simulink model "JetStar_MIL_Simulink"  (R2024b)
settings: Solver=ode4  StartTime=0.0  StopTime=5000  FixedStep=T_Step  RelTol=1e-3
undefined symbols (not defined in the file or in its folder): A_Full_Linear_Long, A_lat, alpha, alpha_calc_rad, alpha_rad, B_Full_Linear_Long, B_lat, beta, beta_rad, C_Full_Linear_Long, C_lat, D_Full_Linear_Long, D_lat, deg, delta_aileron_action_rad, delta_beta_rad, delta_elevator_action_rad, delta_p_radsec, delta_phi_rad, delta_psi_rad, delta_q_radsec, delta_r_radsec, delta_rudder_action_rad, delta_theta_rad, delta_thrust_action_lbs, delta_u, delta_v, delta_w, Earth, ft, g, gamma_calc_rad, H_calc_ft, H_ft, initial, Ixx, Iyy, Izz, m, Matrix_Controls, Matrix_States, p, p_radsec, phi, phi_rad, psi, psi_rad, q, q_radsec, r, r_radsec, rad, RefStates, s, theta, theta_rad, v, V_total, Vehicle, Vtot ... (+9)
libraries: aerolibconvert2 x53, simulink_extras x10, dspsrcs4 x2, aerolibasang x2, aerolibfltsims x2, SignalEditorBlockLib x1, shared6dof x1, dspsigops x1, aerolibtransform2 x1
settings Model: Creator=Abdallah Saleh  LastModifiedBy=mosta

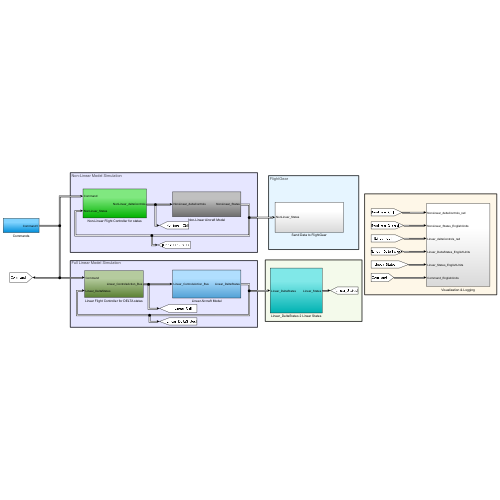
[thumbnail: Simulink's stored preview of the top-level diagram]
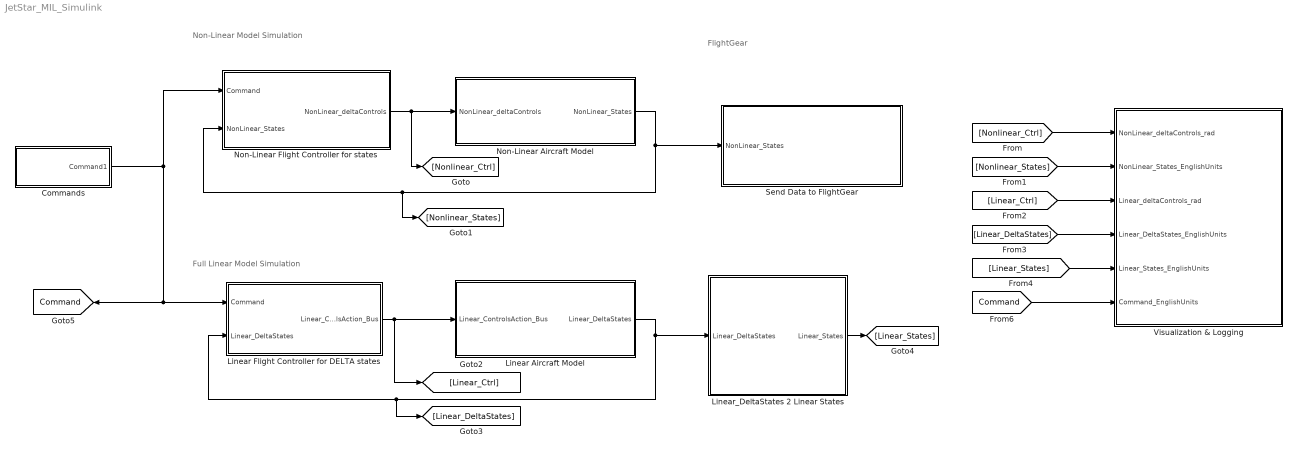
== system JetStar_MIL_Simulink ==
  note: FlightGear
  note: Non-Linear Model Simulation
  note: Full Linear Model Simulation
  Commands : Subsystem
  Linear Aircraft Model : Subsystem
  Linear Flight Controller for DELTA states : Subsystem
  Linear_DeltaStates 2 Linear States : Subsystem
  Non-Linear Aircraft Model : Subsystem
  Non-Linear Flight Controller for states : Subsystem
  Send Data to FlightGear : Subsystem
  Visualization & Logging : Subsystem
  tag scope: Command=global
  wires:
  Non-Linear Flight Controller for states/1(NonLinear_deltaControls) -> [Nonlinear_Ctrl], Non-Linear Aircraft Model/1(NonLinear_deltaControls)
  Non-Linear Aircraft Model/1(NonLinear_States) -> [Nonlinear_States], Non-Linear Flight Controller for states/2(NonLinear_States), Send Data to FlightGear/1(NonLinear_States)
  Linear Flight Controller for DELTA states/1(Linear_ControlsAction_Bus) -> [Linear_Ctrl], Linear Aircraft Model/1(Linear_ControlsAction_Bus)
  Linear Aircraft Model/1(Linear_DeltaStates) -> Linear Flight Controller for DELTA states/2(Linear_DeltaStates), [Linear_DeltaStates], Linear_DeltaStates 2 Linear States/1(Linear_DeltaStates)
  [Nonlinear_Ctrl] -> Visualization & Logging/1(NonLinear_deltaControls_rad)
  [Nonlinear_States] -> Visualization & Logging/2(NonLinear_States_EnglishUnits)
  [Linear_Ctrl] -> Visualization & Logging/3(Linear_deltaControls_rad)
  [Linear_DeltaStates] -> Visualization & Logging/4(Linear_DeltaStates_EnglishUnits)
  Linear_DeltaStates 2 Linear States/1(Linear_States) -> [Linear_States]
  [Linear_States] -> Visualization & Logging/5(Linear_States_EnglishUnits)
  [Command] -> Visualization & Logging/6(Command_EnglishUnits)
  Commands/1(Command1) -> Non-Linear Flight Controller for states/1(Command), Linear Flight Controller for DELTA states/1(Command), [Command]

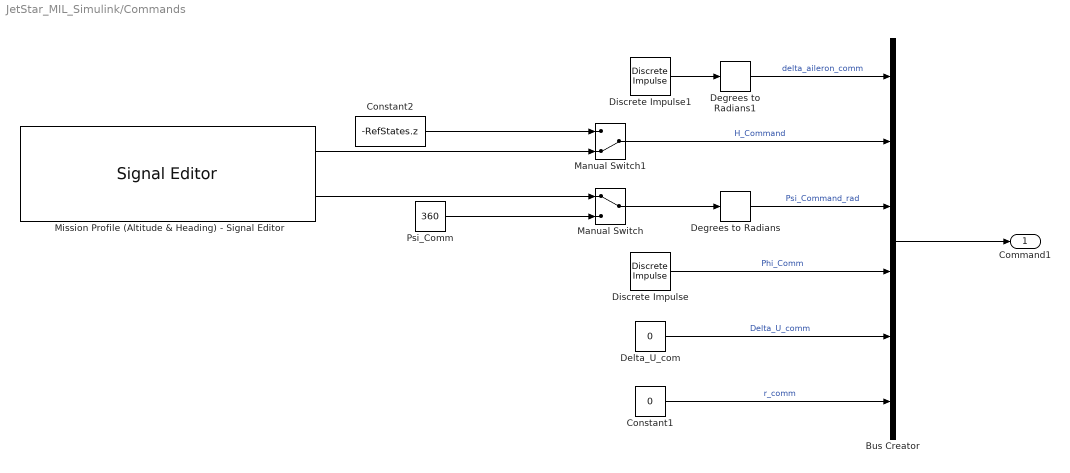
== system JetStar_MIL_Simulink/Commands ==
  Bus Creator : BusCreator  Inputs=6
  Constant1 : Constant  Value=0
  Constant2 : Constant  Value=-RefStates.z
  Degrees to Radians : simulink_extras/Transformations/Degrees to Radians
  Degrees to Radians1 : simulink_extras/Transformations/Degrees to Radians
  Delta_U_com : Constant  Value=0
  Discrete Impulse : dspsrcs4/Discrete  Impulse  Delay=2  SampleTime=15  FrameSample=1  OutputFrames=off  dataType=double  isSigned=on  wordLen=16  udDataType=sfix(16)  fracBitsMode=Best precision  numFracBits=15  OutDataTypeStr=double  LastOutDataTypeStr=double
  Discrete Impulse1 : dspsrcs4/Discrete  Impulse  Delay=1  SampleTime=3  FrameSample=1  OutputFrames=off  dataType=double  isSigned=on  wordLen=16  udDataType=sfix(16)  fracBitsMode=Best precision  numFracBits=15  OutDataTypeStr=double  LastOutDataTypeStr=double
  Manual Switch : ManualSwitch
  Manual Switch1 : ManualSwitch  CurrentSetting=0
  Mission Profile (Altitude & Heading) - Signal Editor : SignalEditorBlockLib/Signal Editor  FileName=Mission_Command.mat  ActiveScenario=Scenario  ActiveSignal=H_mission  IsBus=off  OutputBusObjectStr=Bus: BusObject  SampleTime=0  ZeroCross=off  OutputAfterFinalValue=Setting to zero  Unit=inherit  PreserveSignalName=on  ApplySigPropsToAllScenarios=off  ApplySigPropsToAllSignals=on
  Psi_Comm : Constant  Value=360
  Command1 : Outport
  wires:
  Constant1/1 -> Bus Creator/6  "r_comm"
  Manual Switch1/1 -> Bus Creator/2  "H_Command"
  Degrees to Radians/1 -> Bus Creator/3  "Psi_Command_rad"
  Delta_U_com/1 -> Bus Creator/5  "Delta_U_comm"
  Discrete Impulse/1 -> Bus Creator/4  "Phi_Comm"
  Psi_Comm/1 -> Manual Switch/2
  Manual Switch/1 -> Degrees to Radians/1
  Constant2/1 -> Manual Switch1/1
  Bus Creator/1 -> Command1/1
  Degrees to Radians1/1 -> Bus Creator/1  "delta_aileron_comm"
  Discrete Impulse1/1 -> Degrees to Radians1/1
  Mission Profile (Altitude & Heading) - Signal Editor/2 -> Manual Switch/1
  Mission Profile (Altitude & Heading) - Signal Editor/1 -> Manual Switch1/2

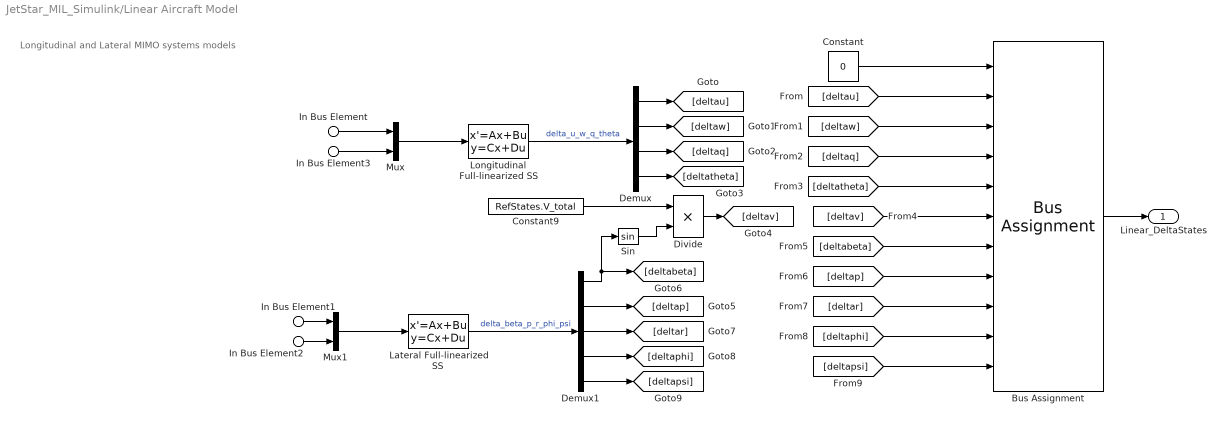
== system JetStar_MIL_Simulink/Linear Aircraft Model ==
  note: Longitudinal and Lateral MIMO systems models
  In Bus Element : Inport  PortName=Linear_ControlsAction_Bus  Element=delta_elevator_action_rad
  In Bus Element1 : Inport  PortName=Linear_ControlsAction_Bus  Element=delta_aileron_action_rad
  In Bus Element2 : Inport  PortName=Linear_ControlsAction_Bus  Element=delta_rudder_action_rad
  In Bus Element3 : Inport  PortName=Linear_ControlsAction_Bus  Element=delta_thrust_action_lbs
  Bus Assignment : BusAssignment  AssignedSignals=delta_u,delta_w,delta_q_radsec,delta_theta_rad,delta_v,delta_beta_rad,delta_p_radsec,delta_r_radsec,delta_phi_rad,delta_psi_rad
  Constant : Constant  Value=0  OutDataTypeStr=Bus: Linear_DeltaStates_Bus
  Constant9 : Constant  Value=RefStates.V_total
  Demux : Demux
  Demux1 : Demux  Outputs=5
  Divide : Product  Inputs=**
  Lateral Full-linearized SS : StateSpace  A=A_lat  B=B_lat  C=C_lat  D=D_lat  InitialCondition=0
  Longitudinal Full-linearized SS : StateSpace  A=A_Full_Linear_Long  B=B_Full_Linear_Long  C=C_Full_Linear_Long  D=D_Full_Linear_Long  InitialCondition=0
  Mux : Mux  Inputs=2
  Mux1 : Mux  Inputs=2
  Sin : Trigonometry
  Linear_DeltaStates : Outport  OutDataTypeStr=Bus: Linear_DeltaStates_Bus
  wires:
  In Bus Element/1 -> Mux/1
  Mux/1 -> Longitudinal Full-linearized SS/1
  In Bus Element3/1 -> Mux/2
  Longitudinal Full-linearized SS/1 -> Demux/1  "delta_u_w_q_theta"
  Mux1/1 -> Lateral Full-linearized SS/1
  Lateral Full-linearized SS/1 -> Demux1/1  "delta_beta_p_r_phi_psi"
  Demux1/1 -> [deltabeta], Sin/1
  In Bus Element2/1 -> Mux1/2
  In Bus Element1/1 -> Mux1/1
  Constant9/1 -> Divide/1
  Sin/1 -> Divide/2
  Constant/1 -> Bus Assignment/1
  Demux/1 -> [deltau]
  Demux/2 -> [deltaw]
  Demux/3 -> [deltaq]
  Demux/4 -> [deltatheta]
  Divide/1 -> [deltav]
  Demux1/2 -> [deltap]
  Demux1/3 -> [deltar]
  Demux1/4 -> [deltaphi]
  Demux1/5 -> [deltapsi]
  [deltau] -> Bus Assignment/2
  [deltaw] -> Bus Assignment/3
  [deltaq] -> Bus Assignment/4
  [deltatheta] -> Bus Assignment/5
  [deltav] -> Bus Assignment/6
  [deltabeta] -> Bus Assignment/7
  [deltap] -> Bus Assignment/8
  [deltar] -> Bus Assignment/9
  [deltaphi] -> Bus Assignment/10
  [deltapsi] -> Bus Assignment/11
  Bus Assignment/1 -> Linear_DeltaStates/1

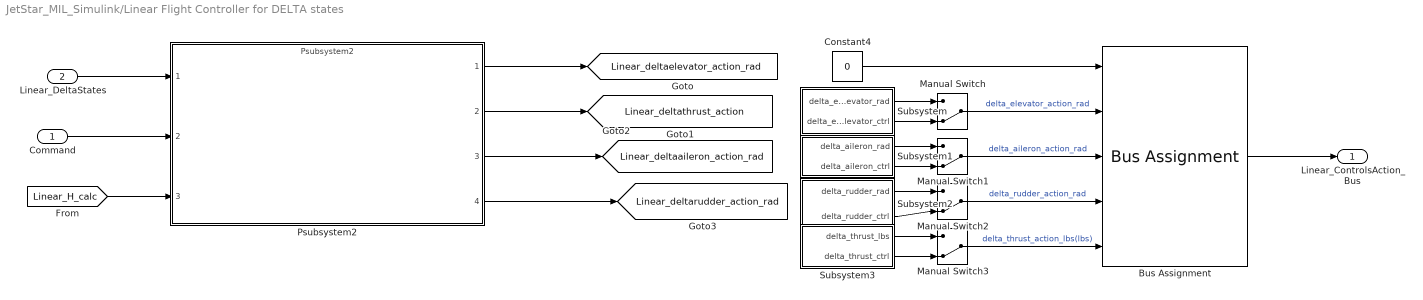
== system JetStar_MIL_Simulink/Linear Flight Controller for DELTA states ==
  Command : Inport
  Linear_DeltaStates : Inport  Port=2
  Bus Assignment : BusAssignment  AssignedSignals=delta_elevator_action_rad,delta_aileron_action_rad,delta_rudder_action_rad,delta_thrust_action_lbs
  Constant4 : Constant  Value=0  OutDataTypeStr=Bus: Linear_ControlsAction_Bus
  Manual Switch{,1..3} (4 alike) : ManualSwitch  CurrentSetting=0
  Psubsystem2 : ModelReference  ModelNameDialog=Psubsystem2  ModelReferenceVersion=1.395  CopyOfModelProtected=on
  Subsystem : Subsystem
  Subsystem1 : Subsystem
  Subsystem2 : Subsystem
  Subsystem3 : Subsystem
  Linear_ControlsAction_Bus : Outport  OutDataTypeStr=Bus: Linear_ControlsAction_Bus
  tag scope: Linear_deltaaileron_action_rad=global, Linear_deltaelevator_action_rad=global, Linear_deltarudder_action_rad=global, Linear_deltathrust_action=global
  wires:
  Constant4/1 -> Bus Assignment/1
  Manual Switch/1 -> Bus Assignment/2  "delta_elevator_action_rad"
  Manual Switch1/1 -> Bus Assignment/3  "delta_aileron_action_rad"
  Manual Switch2/1 -> Bus Assignment/4  "delta_rudder_action_rad"
  Manual Switch3/1 -> Bus Assignment/5  "delta_thrust_action_lbs(lbs)"
  Bus Assignment/1 -> Linear_ControlsAction_Bus/1
  Subsystem/1(delta_elevator_rad) -> Manual Switch/1
  Subsystem/2(delta_elevator_ctrl) -> Manual Switch/2
  Subsystem1/1(delta_aileron_rad) -> Manual Switch1/1
  Subsystem1/2(delta_aileron_ctrl) -> Manual Switch1/2
  Subsystem2/1(delta_rudder_rad) -> Manual Switch2/1
  Subsystem2/2(delta_rudder_ctrl) -> Manual Switch2/2
  Subsystem3/1(delta_thrust_lbs) -> Manual Switch3/1
  Subsystem3/2(delta_thrust_ctrl) -> Manual Switch3/2
  Linear_DeltaStates/1 -> Psubsystem2/1
  [Linear_H_calc] -> Psubsystem2/3
  Command/1 -> Psubsystem2/2
  Psubsystem2/1 -> [Linear_deltaelevator_action_rad]
  Psubsystem2/2 -> [Linear_deltathrust_action]
  Psubsystem2/3 -> [Linear_deltaaileron_action_rad]
  Psubsystem2/4 -> [Linear_deltarudder_action_rad]

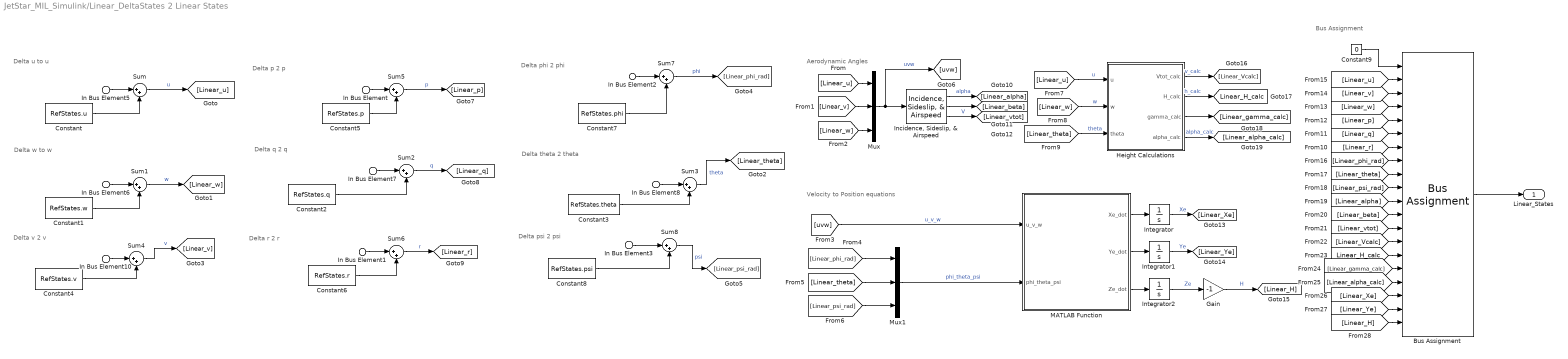
== system JetStar_MIL_Simulink/Linear_DeltaStates 2 Linear States ==
  note: Bus Assignment
  note: Velocity to Position equations
  note: Aerodynamic Angles
  note: Delta psi 2 psi
  note: Delta phi 2 phi
  note: Delta r 2 r
  note: Delta p 2 p
  note: Delta v 2 v
  note: Delta theta 2 theta
  note: Delta q 2 q
  note: Delta w to w
  note: Delta u to u
  In Bus Element : Inport  PortName=Linear_DeltaStates  Element=delta_p_radsec
  In Bus Element1 : Inport  PortName=Linear_DeltaStates  Element=delta_r_radsec
  In Bus Element2 : Inport  PortName=Linear_DeltaStates  Element=delta_phi_rad
  In Bus Element3 : Inport  PortName=Linear_DeltaStates  Element=delta_psi_rad
  In Bus Element5 : Inport  PortName=Linear_DeltaStates  Element=delta_u
  In Bus Element6 : Inport  PortName=Linear_DeltaStates  Element=delta_w
  In Bus Element7 : Inport  PortName=Linear_DeltaStates  Element=delta_q_radsec
  In Bus Element8 : Inport  PortName=Linear_DeltaStates  Element=delta_theta_rad
  In Bus Element10 : Inport  PortName=Linear_DeltaStates  Element=delta_v
  Bus Assignment : BusAssignment  AssignedSignals=u,v,w,p_radsec,q_radsec,r_radsec,phi_rad,theta_rad,psi_rad,alpha_rad,beta_rad,Vtot,Vtot_calc,H_calc_ft,gamma_calc_rad,alpha_calc_rad,Xe_ft,Ye_ft,H_ft
  Constant : Constant  Value=RefStates.u
  Constant1 : Constant  Value=RefStates.w
  Constant2 : Constant  Value=RefStates.q
  Constant3 : Constant  Value=RefStates.theta
  Constant4 : Constant  Value=RefStates.v
  Constant5 : Constant  Value=RefStates.p
  Constant6 : Constant  Value=RefStates.r
  Constant7 : Constant  Value=RefStates.phi
  Constant8 : Constant  Value=RefStates.psi
  Constant9 : Constant  Value=0  OutDataTypeStr=Bus: Linear_States_Bus
  Gain : Gain  Gain=-1
  Height Calculations : Subsystem
  "Incidence, Sideslip, & Airspeed" : aerolibasang/Incidence, Sideslip, & Airspeed
  Integrator : Integrator
  Integrator1 : Integrator
  Integrator2 : Integrator
  MATLAB Function : MATLAB Function  TreatAsAtomicUnit=on
  Mux : Mux  Inputs=3
  Mux1 : Mux  Inputs=3
  Sum{,1..8} (9 alike) : Sum  Inputs=|++
  Linear_States : Outport  OutDataTypeStr=Bus: Linear_States_Bus
  tag scope: Linear_H_calc=global
  wires:
  In Bus Element5/1 -> Sum/1
  Constant/1 -> Sum/2
  Sum/1 -> [Linear_u]  "u"
  In Bus Element6/1 -> Sum1/1
  Constant1/1 -> Sum1/2
  Sum1/1 -> [Linear_w]  "w"
  In Bus Element7/1 -> Sum2/1
  Constant2/1 -> Sum2/2
  Sum2/1 -> [Linear_q]  "q"
  In Bus Element8/1 -> Sum3/1
  Constant3/1 -> Sum3/2
  Sum3/1 -> [Linear_theta]  "theta"
  Constant4/1 -> Sum4/2
  Sum4/1 -> [Linear_v]  "v"
  In Bus Element/1 -> Sum5/1
  Constant5/1 -> Sum5/2
  Sum5/1 -> [Linear_p]  "p"
  In Bus Element1/1 -> Sum6/1
  Sum6/1 -> [Linear_r]  "r"
  Constant6/1 -> Sum6/2
  In Bus Element2/1 -> Sum7/1
  Constant7/1 -> Sum7/2
  Sum7/1 -> [Linear_phi_rad]  "phi"
  In Bus Element3/1 -> Sum8/1
  Constant8/1 -> Sum8/2
  Sum8/1 -> [Linear_psi_rad]  "psi"
  Mux/1 -> [uvw], "Incidence, Sideslip, & Airspeed"/1  "uvw"
  [Linear_u] -> Mux/1
  [Linear_v] -> Mux/2
  [Linear_w] -> Mux/3
  [Linear_phi_rad] -> Mux1/1
  [Linear_theta] -> Mux1/2
  [Linear_psi_rad] -> Mux1/3
  Mux1/1 -> MATLAB Function/2(phi_theta_psi)  "phi_theta_psi"
  In Bus Element10/1 -> Sum4/1
  [uvw] -> MATLAB Function/1(u_v_w)  "u_v_w"
  MATLAB Function/1(Xe_dot) -> Integrator/1
  MATLAB Function/2(Ye_dot) -> Integrator1/1
  MATLAB Function/3(Ze_dot) -> Integrator2/1
  Integrator2/1 -> Gain/1  "Ze"
  Gain/1 -> [Linear_H]  "H"
  [Linear_u] -> Height Calculations/1(u)  "u"
  [Linear_w] -> Height Calculations/2(w)  "w"
  [Linear_theta] -> Height Calculations/3(theta)  "theta"
  Height Calculations/1(Vtot_calc) -> [Linear_Vcalc]  "v_calc"
  Height Calculations/2(H_calc) -> [Linear_H_calc]  "h_calc"
  Height Calculations/3(gamma_calc) -> [Linear_gamma_calc]
  "Incidence, Sideslip, & Airspeed"/1 -> [Linear_alpha]  "alpha"
  "Incidence, Sideslip, & Airspeed"/2 -> [Linear_beta]
  "Incidence, Sideslip, & Airspeed"/3 -> [Linear_vtot]  "V"
  Integrator/1 -> [Linear_Xe]  "Xe"
  Integrator1/1 -> [Linear_Ye]  "Ye"
  Height Calculations/4(alpha_calc) -> [Linear_alpha_calc]  "alpha_calc"
  [Linear_u] -> Bus Assignment/2
  [Linear_v] -> Bus Assignment/3
  [Linear_w] -> Bus Assignment/4
  [Linear_p] -> Bus Assignment/5
  [Linear_q] -> Bus Assignment/6
  [Linear_r] -> Bus Assignment/7
  [Linear_phi_rad] -> Bus Assignment/8
  [Linear_theta] -> Bus Assignment/9
  [Linear_psi_rad] -> Bus Assignment/10
  [Linear_alpha] -> Bus Assignment/11
  [Linear_beta] -> Bus Assignment/12
  [Linear_vtot] -> Bus Assignment/13
  [Linear_Vcalc] -> Bus Assignment/14
  [Linear_H_calc] -> Bus Assignment/15
  [Linear_Xe] -> Bus Assignment/18
  [Linear_Ye] -> Bus Assignment/19
  [Linear_H] -> Bus Assignment/20
  [Linear_gamma_calc] -> Bus Assignment/16
  [Linear_alpha_calc] -> Bus Assignment/17
  Constant9/1 -> Bus Assignment/1
  Bus Assignment/1 -> Linear_States/1

== system JetStar_MIL_Simulink/Non-Linear Aircraft Model ==
  NonLinear_deltaControls : Inport  OutDataTypeStr=Bus: Nonlinear_ControlsAction_Bus
  Airframe_Model : Subsystem
  Delay1 : Delay  DelayLength=1  InitialCondition=RefStates
  Euler_6DOF : Subsystem
  NonLinear_States : Outport  OutDataTypeStr=Bus: Nonlinear_States_Bus
  wires:
  NonLinear_deltaControls/1 -> Airframe_Model/2(NonLinear_deltaControls)
  Delay1/1 -> Airframe_Model/1(StatesBus)
  Airframe_Model/1(Forces) -> Euler_6DOF/1(Forces)
  Airframe_Model/2(Moments) -> Euler_6DOF/2(Moments)
  Euler_6DOF/1(States) -> Delay1/1, NonLinear_States/1

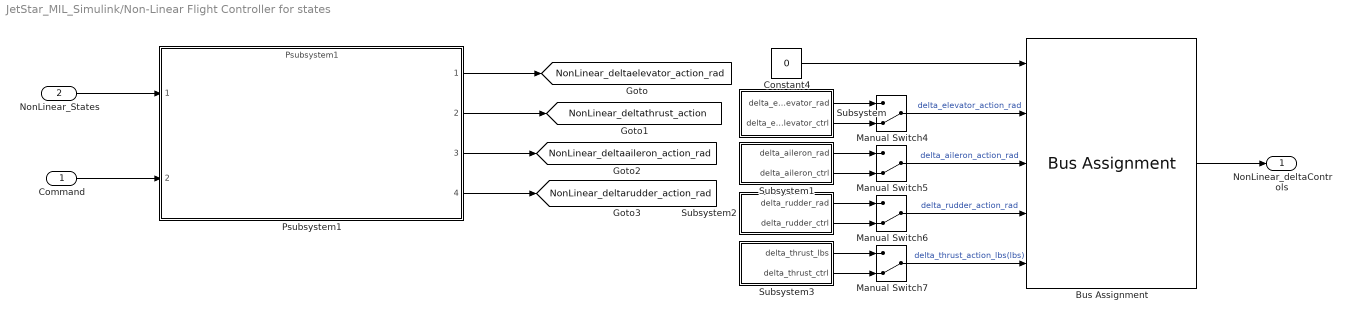
== system JetStar_MIL_Simulink/Non-Linear Flight Controller for states ==
  Command : Inport
  NonLinear_States : Inport  Port=2
  Bus Assignment : BusAssignment  AssignedSignals=delta_elevator_action_rad,delta_aileron_action_rad,delta_rudder_action_rad,delta_thrust_action_lbs
  Constant4 : Constant  Value=0  OutDataTypeStr=Bus: Nonlinear_ControlsAction_Bus
  Manual Switch{4..7} (4 alike) : ManualSwitch  CurrentSetting=0
  Psubsystem1 : ModelReference  ModelNameDialog=Psubsystem1  ModelReferenceVersion=1.395  CopyOfModelProtected=on
  Subsystem : Subsystem
  Subsystem1 : Subsystem
  Subsystem2 : Subsystem
  Subsystem3 : Subsystem
  NonLinear_deltaControls : Outport  OutDataTypeStr=Bus: Nonlinear_ControlsAction_Bus
  tag scope: NonLinear_deltaaileron_action_rad=global, NonLinear_deltaelevator_action_rad=global, NonLinear_deltarudder_action_rad=global, NonLinear_deltathrust_action=global
  wires:
  Constant4/1 -> Bus Assignment/1
  Bus Assignment/1 -> NonLinear_deltaControls/1
  Subsystem2/1(delta_rudder_rad) -> Manual Switch6/1
  Subsystem2/2(delta_rudder_ctrl) -> Manual Switch6/2
  Subsystem3/1(delta_thrust_lbs) -> Manual Switch7/1
  Subsystem3/2(delta_thrust_ctrl) -> Manual Switch7/2
  Subsystem/2(delta_elevator_ctrl) -> Manual Switch4/2
  Subsystem/1(delta_elevator_rad) -> Manual Switch4/1
  Subsystem1/2(delta_aileron_ctrl) -> Manual Switch5/2
  Manual Switch6/1 -> Bus Assignment/4  "delta_rudder_action_rad"
  Manual Switch5/1 -> Bus Assignment/3  "delta_aileron_action_rad"
  Manual Switch7/1 -> Bus Assignment/5  "delta_thrust_action_lbs(lbs)"
  Manual Switch4/1 -> Bus Assignment/2  "delta_elevator_action_rad"
  Subsystem1/1(delta_aileron_rad) -> Manual Switch5/1
  NonLinear_States/1 -> Psubsystem1/1
  Command/1 -> Psubsystem1/2
  Psubsystem1/1 -> [NonLinear_deltaelevator_action_rad]
  Psubsystem1/2 -> [NonLinear_deltathrust_action]
  Psubsystem1/3 -> [NonLinear_deltaaileron_action_rad]
  Psubsystem1/4 -> [NonLinear_deltarudder_action_rad]

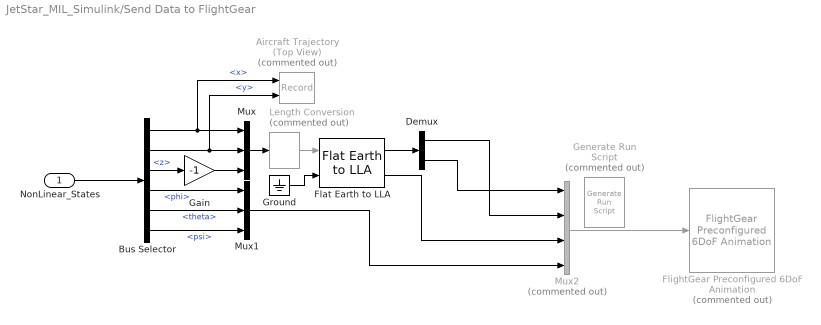
== system JetStar_MIL_Simulink/Send Data to FlightGear ==
  NonLinear_States : Inport  OutDataTypeStr=Bus: Nonlinear_States_Bus
  Aircraft Trajectory (Top View) : Record  Commented=on  FileSettingsInternal="{\"entries\":[{\"content\":{\"excelSettings\":{\"content\":{},\"type\":\"Streamout.ExcelSettings\"}},\"type\":\"Streamout.FileSettingStorage\",\"uuid\":\"\"}],\"packageUris\":[\"http:\\/\\/schema.mathworks.com\\/mf0\\/streamout_blocks\\/R2020a\"],\"version\":\"1.0\"}"  Layout=[1 1]  SignalsInternal="{\"entries\":[{\"content\":{},\"type\":\"RecordBlkView.InputSignals\",\"uuid\":\"\"}],\"packageUris\":[\"http:\\/\\/schema.mathworks.com\\/mf0\\/streamout_blocks\\/R2020a\"],\"version\":\"1.0\"}"  VisualizationBindings="{\"xyplotplugin\":{\"info\":[{\"series\":[],\"subplotID\":1}]}}"  CompatibilityTag=XY
  Bus Selector : BusSelector  OutputSignals=x,y,z,phi,theta,psi
  Demux : Demux  Outputs=2
  Flat Earth to LLA : aerolibtransform2/Flat Earth to LLA  units=Metric (MKS)  ptype=Earth (WGS84)  F=1/298.257223563  R=6378137  refPosPort=off  LL0=[0 10]  psi=0
  FlightGear Preconfigured 6DoF Animation : aerolibfltsims/FlightGear Preconfigured 6DoF Animation  Commented=on  xFlightGearVersion=v2019.1  DestinationIpAddress=127.0.0.1  DestinationPort=5502  SampleTime=-1  packetVersion=24
  Gain : Gain  Gain=-1
  Generate Run Script : aerolibfltsims/Generate Run Script  Commented=on  Architecture=Win64  dataFlow=Send  GeometryModelName=HL20  AirportId=KSFO  RunwayId=10L  InitialAltitude=0  InitialHeading=0  OffsetDistance=0  OffsetAzimuth=0  InstallScenery=off  DisableShaders=on  OriginAddress=127.0.0.1  DestinationPort=5502  OriginPort=5505  LocalAddress=127.0.0.1  OutputFileName=runfg.bat  FlightGearBaseDirectory=C:\Program Files\FlightGear 2024.1
  Ground : Ground
  Length Conversion : aerolibconvert2/Length Conversion  Commented=on  IU=ft  OU=m
  Mux : Mux  Inputs=3
  Mux1 : Mux  Inputs=3
  Mux2 : Mux  Commented=on
  wires:
  NonLinear_States/1 -> Bus Selector/1
  Bus Selector/1 -> Mux/1, Aircraft Trajectory (Top View)/1  "<x>"
  Bus Selector/2 -> Mux/2, Aircraft Trajectory (Top View)/2  "<y>"
  Bus Selector/3 -> Gain/1  "<z>"
  Bus Selector/4 -> Mux1/1  "<phi>"
  Bus Selector/5 -> Mux1/2  "<theta>"
  Bus Selector/6 -> Mux1/3  "<psi>"
  Mux/1 -> Length Conversion/1
  Ground/1 -> Flat Earth to LLA/2
  Mux2/1 -> FlightGear Preconfigured 6DoF Animation/1
  Flat Earth to LLA/1 -> Demux/1
  Demux/1 -> Mux2/2
  Demux/2 -> Mux2/1
  Mux1/1 -> Mux2/4
  Flat Earth to LLA/2 -> Mux2/3
  Length Conversion/1 -> Flat Earth to LLA/1
  Gain/1 -> Mux/3

== system JetStar_MIL_Simulink/Visualization & Logging ==
  NonLinear_deltaControls_rad : Inport
  NonLinear_States_EnglishUnits : Inport  Port=2
  Linear_deltaControls_rad : Inport  Port=3
  Linear_DeltaStates_EnglishUnits : Inport  Port=4
  Linear_States_EnglishUnits : Inport  Port=5
  Command_EnglishUnits : Inport  Port=6
  Units conversion & Data logging : Subsystem
  Units conversion & Data logging1 : Subsystem
  Units conversion & Data logging2 : Subsystem
  Units conversion & Data logging3 : Subsystem
  Units conversion & Data logging4 : Subsystem
  Units conversion & Data logging5 : Subsystem
  wires:
  NonLinear_States_EnglishUnits/1 -> Units conversion & Data logging1/1(NonLinear_States_EnglishUnits)  "NonLinear_States_EnglishUnits"
  Linear_deltaControls_rad/1 -> Units conversion & Data logging2/1(Linear_deltaControls_rad)  "Linear_deltaControls_rad"
  Linear_DeltaStates_EnglishUnits/1 -> Units conversion & Data logging3/1(Linear_DeltaStates_EnglishUnits)  "Linear_DeltaStates_EnglishUnits"
  Linear_States_EnglishUnits/1 -> Units conversion & Data logging4/1(Linear_States_EnglishUnits)  "Linear_States_EnglishUnits"
  NonLinear_deltaControls_rad/1 -> Units conversion & Data logging/1(NonLinear_deltaControls_rad)  "NonLinear_deltaControls_rad"
  Command_EnglishUnits/1 -> Units conversion & Data logging5/1(Command_EnglishUnits)  "Command_EnglishUnits"

== system JetStar_MIL_Simulink/Linear Flight Controller for DELTA states/Subsystem ==
  Constant : Constant  Value=0
  Degrees to Radians : simulink_extras/Transformations/Degrees to Radians
  delta_elevator_rad : Outport
  delta_elevator_ctrl : Outport  Port=2
  wires:
  [Linear_deltaelevator_action_rad] -> delta_elevator_ctrl/1  "delta_elevator_ctrl"
  Constant/1 -> Degrees to Radians/1
  Degrees to Radians/1 -> delta_elevator_rad/1  "delta_elevator_rad"

== system JetStar_MIL_Simulink/Linear Flight Controller for DELTA states/Subsystem1 ==
  Constant1 : Constant  Value=0
  Degrees to Radians1 : simulink_extras/Transformations/Degrees to Radians
  delta_aileron_rad : Outport
  delta_aileron_ctrl : Outport  Port=2
  wires:
  Constant1/1 -> Degrees to Radians1/1
  [Linear_deltaaileron_action_rad] -> delta_aileron_ctrl/1  "delta_aileron_ctrl"
  Degrees to Radians1/1 -> delta_aileron_rad/1  "delta_aileron_rad"

== system JetStar_MIL_Simulink/Linear Flight Controller for DELTA states/Subsystem2 ==
  Constant2 : Constant  Value=0
  Degrees to Radians2 : simulink_extras/Transformations/Degrees to Radians
  delta_rudder_rad : Outport
  delta_rudder_ctrl : Outport  Port=2
  wires:
  Constant2/1 -> Degrees to Radians2/1
  [Linear_deltarudder_action_rad] -> delta_rudder_ctrl/1  "delta_rudder_ctrl"
  Degrees to Radians2/1 -> delta_rudder_rad/1  "delta_rudder_rad"

== system JetStar_MIL_Simulink/Linear Flight Controller for DELTA states/Subsystem3 ==
  Constant3 : Constant  Value=0
  delta_thrust_lbs : Outport
  delta_thrust_ctrl : Outport  Port=2
  wires:
  [Linear_deltathrust_action] -> delta_thrust_ctrl/1  "delta_thrust_ctrl"
  Constant3/1 -> delta_thrust_lbs/1  "delta_thrust_lbs"

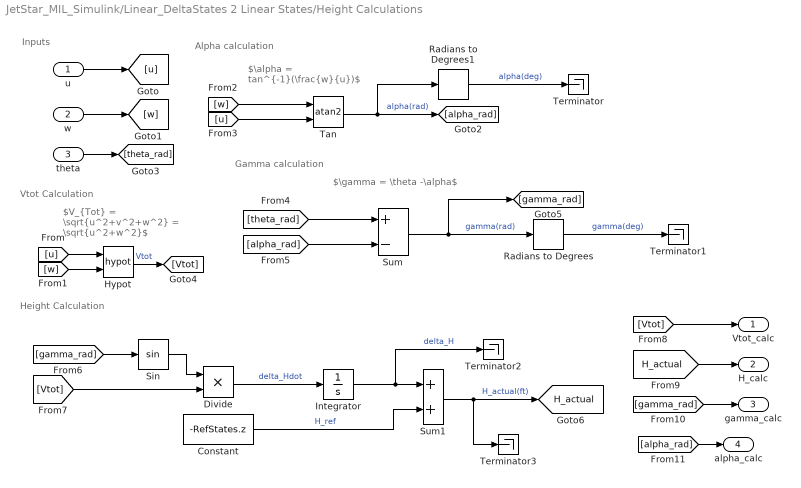
== system JetStar_MIL_Simulink/Linear_DeltaStates 2 Linear States/Height Calculations ==
  note: Gamma calculation
  note: $\alpha = tan^{-1}(\frac{w}{u})$
  note: Alpha calculation
  note: Inputs
  note: Height Calculation
  note: $V_{Tot} = \sqrt{u^2+v^2+w^2} = \sqrt{u^2+w^2}$
  note: $\gamma = \theta -\alpha$
  note: Vtot Calculation
  u : Inport
  w : Inport  Port=2
  theta : Inport  Port=3
  Constant : Constant  Value=-RefStates.z
  Divide : Product  Inputs=**
  Hypot : Math  Operator=hypot
  Integrator : Integrator
  Radians to Degrees : simulink_extras/Transformations/Radians to Degrees
  Radians to Degrees1 : simulink_extras/Transformations/Radians to Degrees
  Sin : Trigonometry
  Sum : Sum  Inputs=+-
  Sum1 : Sum
  Tan : Trigonometry  Operator=atan2
  Terminator{,1..3} (4 alike) : Terminator
  Vtot_calc : Outport
  H_calc : Outport  Port=2
  gamma_calc : Outport  Port=3
  alpha_calc : Outport  Port=4
  tag scope: H_actual=global
  wires:
  Sum/1 -> [gamma_rad], Radians to Degrees/1  "gamma(rad)"
  Sum1/1 -> Terminator3/1, [H_actual]  "H_actual(ft)"
  Hypot/1 -> [Vtot]  "Vtot"
  [theta_rad] -> Sum/1
  [u] -> Tan/2
  Constant/1 -> Sum1/2  "H_ref"
  Divide/1 -> Integrator/1  "delta_Hdot"
  [u] -> Hypot/1
  theta/1 -> [theta_rad]
  [Vtot] -> Divide/2
  Tan/1 -> Radians to Degrees1/1, [alpha_rad]  "alpha(rad)"
  [gamma_rad] -> Sin/1
  Radians to Degrees/1 -> Terminator1/1  "gamma(deg)"
  Integrator/1 -> Terminator2/1, Sum1/1  "delta_H"
  Sin/1 -> Divide/1
  [w] -> Tan/1
  [alpha_rad] -> Sum/2
  [w] -> Hypot/2
  u/1 -> [u]
  w/1 -> [w]
  Radians to Degrees1/1 -> Terminator/1  "alpha(deg)"
  [Vtot] -> Vtot_calc/1
  [H_actual] -> H_calc/1
  [gamma_rad] -> gamma_calc/1
  [alpha_rad] -> alpha_calc/1

== system JetStar_MIL_Simulink/Non-Linear Aircraft Model/Airframe_Model ==
  StatesBus : Inport
  NonLinear_deltaControls : Inport  Port=2
  Deltas Forces and Moments : Subsystem
  "Intertias gain " : Gain  Gain=[Ixx;Iyy;Izz]
  "Mass gain " : Gain  Gain=Vehicle.Airframe.mass
  ReferenceForces : Constant  Value=initial.forces  VectorParams1D=off
  ReferenceMoments : Constant  Value=initial.moments
  Sum : Sum  Inputs=|++
  "Sum " : Sum
  Forces : Outport
  Moments : Outport  Port=2
  wires:
  ReferenceMoments/1 -> Sum/2
  Deltas Forces and Moments/2(DeltaMoments) -> "Intertias gain "/1
  Deltas Forces and Moments/1(DeltaForces) -> "Mass gain "/1
  StatesBus/1 -> Deltas Forces and Moments/1(StatesBus)
  Sum/1 -> Moments/1
  ReferenceForces/1 -> "Sum "/1
  "Intertias gain "/1 -> Sum/1
  "Mass gain "/1 -> "Sum "/2
  NonLinear_deltaControls/1 -> Deltas Forces and Moments/2(NonLinear_deltaControls)
  "Sum "/1 -> Forces/1

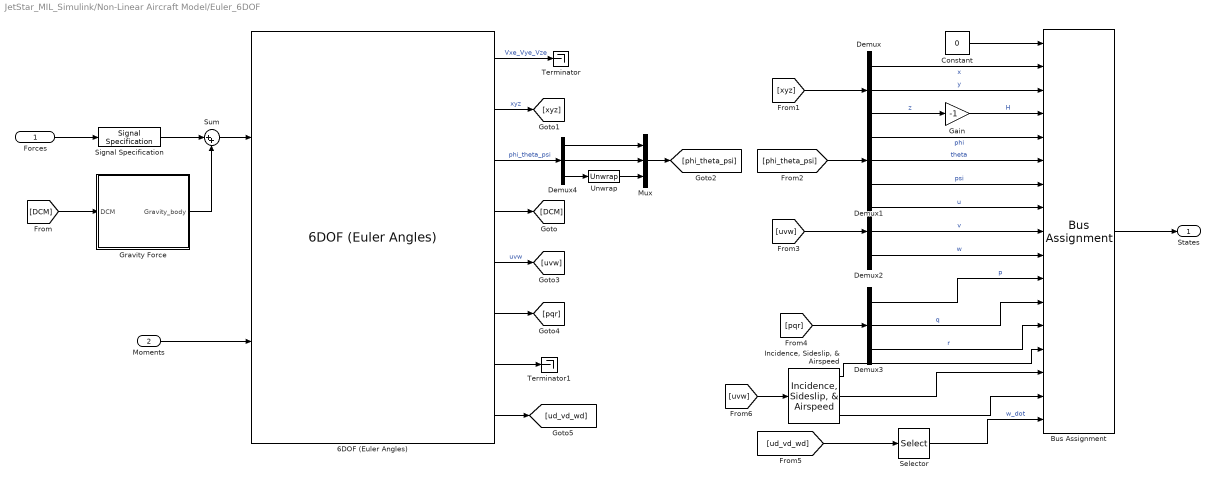
== system JetStar_MIL_Simulink/Non-Linear Aircraft Model/Euler_6DOF ==
  Forces : Inport
  Moments : Inport  Port=2
  6DOF (Euler Angles) : shared6dof/6DOF (Euler Angles)  units=English (Velocity in ft/s)  mtype=Fixed  rep=Euler Angles  xme_0=initial.position  Vm_0=initial.Vbody  eul_0=initial.Euler_Angles  pm_0=initial.AngRates  mass_0=Vehicle.Airframe.mass  mass_e=0.5  mass_f=2.0  inertia=Vehicle.Airframe.inertias  inertia_e=eye(3)  inertia_f=2*eye(3)  k_quat=1.0  vre_flag=on  abi_flag=off  aMode=0  xme_statename=''  Vm_statename=''  eul_statename=''  quat_statename=''  pm_statename=''  mass_statename=''
  Bus Assignment : BusAssignment  AssignedSignals=x,y,z,phi,theta,psi,u,v,w,p,q,r,alpha,beta,V_total,w_dot
  Constant : Constant  Value=0  OutDataTypeStr=Bus: Nonlinear_States_Bus
  Demux{,1..4} (5 alike) : Demux  Outputs=3
  Gain : Gain  Gain=-1
  Gravity Force : Subsystem
  "Incidence, Sideslip, & Airspeed" : aerolibasang/Incidence, Sideslip, & Airspeed
  Mux : Mux  Inputs=3
  Selector : Selector  InputPortWidth=3  IndexOptions=Index vector (dialog)  Indices=[3]  OutputSizes=1
  Signal Specification : SignalSpecification  Dimensions=[3 1]
  Sum : Sum  Inputs=|++
  Terminator : Terminator
  Terminator1 : Terminator
  Unwrap : dspsigops/Unwrap  tol=pi  InputProcessing=Columns as channels (frame based)  running=off
  States : Outport  OutDataTypeStr=Bus: Nonlinear_States_Bus
  wires:
  6DOF (Euler Angles)/8 -> [ud_vd_wd]
  6DOF (Euler Angles)/4 -> [DCM]
  Constant/1 -> Bus Assignment/1
  Moments/1 -> 6DOF (Euler Angles)/2
  Bus Assignment/1 -> States/1
  6DOF (Euler Angles)/1 -> Terminator/1  "Vxe_Vye_Vze"
  6DOF (Euler Angles)/2 -> [xyz]  "xyz"
  [xyz] -> Demux/1
  Demux/1 -> Bus Assignment/2  "x"
  Demux/2 -> Bus Assignment/3  "y"
  Demux/3 -> Gain/1  "z"
  [phi_theta_psi] -> Demux1/1
  Demux1/1 -> Bus Assignment/5  "phi"
  Demux1/2 -> Bus Assignment/6  "theta"
  Demux1/3 -> Bus Assignment/7  "psi"
  Demux2/1 -> Bus Assignment/8  "u"
  Demux2/2 -> Bus Assignment/9  "v"
  6DOF (Euler Angles)/5 -> [uvw]  "uvw"
  [uvw] -> Demux2/1
  6DOF (Euler Angles)/6 -> [pqr]
  [pqr] -> Demux3/1
  6DOF (Euler Angles)/7 -> Terminator1/1
  [uvw] -> "Incidence, Sideslip, & Airspeed"/1
  [ud_vd_wd] -> Selector/1
  [DCM] -> Gravity Force/1(DCM)
  Sum/1 -> 6DOF (Euler Angles)/1
  Forces/1 -> Signal Specification/1
  Gravity Force/1(Gravity_body) -> Sum/2
  Signal Specification/1 -> Sum/1
  Demux2/3 -> Bus Assignment/10  "w"
  Demux3/1 -> Bus Assignment/11  "p"
  Demux3/2 -> Bus Assignment/12  "q"
  Demux3/3 -> Bus Assignment/13  "r"
  "Incidence, Sideslip, & Airspeed"/1 -> Bus Assignment/14
  "Incidence, Sideslip, & Airspeed"/2 -> Bus Assignment/15
  "Incidence, Sideslip, & Airspeed"/3 -> Bus Assignment/16
  Selector/1 -> Bus Assignment/17  "w_dot"
  Gain/1 -> Bus Assignment/4  "H"
  6DOF (Euler Angles)/3 -> Demux4/1  "phi_theta_psi"
  Demux4/3 -> Unwrap/1
  Demux4/1 -> Mux/1
  Demux4/2 -> Mux/2
  Unwrap/1 -> Mux/3
  Mux/1 -> [phi_theta_psi]

== system JetStar_MIL_Simulink/Non-Linear Flight Controller for states/Subsystem ==
  Constant : Constant  Value=0
  Degrees to Radians : simulink_extras/Transformations/Degrees to Radians
  delta_elevator_rad : Outport
  delta_elevator_ctrl : Outport  Port=2
  wires:
  [NonLinear_deltaelevator_action_rad] -> delta_elevator_ctrl/1  "delta_elevator_ctrl"
  Constant/1 -> Degrees to Radians/1
  Degrees to Radians/1 -> delta_elevator_rad/1  "delta_elevator_rad"

== system JetStar_MIL_Simulink/Non-Linear Flight Controller for states/Subsystem1 ==
  Constant1 : Constant  Value=0
  Degrees to Radians1 : simulink_extras/Transformations/Degrees to Radians
  delta_aileron_rad : Outport
  delta_aileron_ctrl : Outport  Port=2
  wires:
  Constant1/1 -> Degrees to Radians1/1
  [NonLinear_deltaaileron_action_rad] -> delta_aileron_ctrl/1  "delta_aileron_ctrl"
  Degrees to Radians1/1 -> delta_aileron_rad/1  "delta_aileron_rad"

== system JetStar_MIL_Simulink/Non-Linear Flight Controller for states/Subsystem2 ==
  Constant2 : Constant  Value=0
  Degrees to Radians2 : simulink_extras/Transformations/Degrees to Radians
  delta_rudder_rad : Outport
  delta_rudder_ctrl : Outport  Port=2
  wires:
  Constant2/1 -> Degrees to Radians2/1
  [NonLinear_deltarudder_action_rad] -> delta_rudder_ctrl/1  "delta_rudder_ctrl"
  Degrees to Radians2/1 -> delta_rudder_rad/1  "delta_rudder_rad"

== system JetStar_MIL_Simulink/Non-Linear Flight Controller for states/Subsystem3 ==
  Constant3 : Constant  Value=0
  delta_thrust_lbs : Outport
  delta_thrust_ctrl : Outport  Port=2
  wires:
  [NonLinear_deltathrust_action] -> delta_thrust_ctrl/1  "delta_thrust_ctrl"
  Constant3/1 -> delta_thrust_lbs/1  "delta_thrust_lbs"

== system JetStar_MIL_Simulink/Visualization & Logging/Units conversion & Data logging ==
  NonLinear_deltaControls_rad : Inport
  Angle Conversion : aerolibconvert2/Angle Conversion  IU=rad  OU=deg
  Angle Conversion1 : aerolibconvert2/Angle Conversion  IU=rad  OU=deg
  Angle Conversion2 : aerolibconvert2/Angle Conversion  IU=rad  OU=deg
  Bus Creator : BusCreator  Inputs=2
  Bus Creator1 : BusCreator  Inputs=4
  Bus Selector : BusSelector  OutputSignals=delta_rudder_action_rad,delta_aileron_action_rad,delta_elevator_action_rad,delta_thrust_action_lbs
  Gain : Gain
  Terminator : Terminator
  To Workspace : ToWorkspace  VariableName=NonLinear_deltaControls  SaveFormat=Timeseries  SampleTime=-1
  wires:
  Angle Conversion2/1 -> Bus Creator1/3  "delta_elevator_action_deg"
  NonLinear_deltaControls_rad/1 -> Bus Selector/1, Bus Creator/2  "NonLinear_deltaControls_rad_lbs"
  Angle Conversion1/1 -> Bus Creator1/2  "delta_aileron_action_deg"
  Angle Conversion/1 -> Bus Creator1/1  "delta_rudder_action_deg"
  Bus Selector/1 -> Angle Conversion/1  "<delta_rudder_action_rad>"
  Bus Selector/4 -> Gain/1  "<delta_thrust_action_lbs>"
  Bus Creator/1 -> To Workspace/1, Terminator/1  "NonLinear_deltaControls"
  Gain/1 -> Bus Creator1/4  "delta_thrust_action_lbs"
  Bus Selector/2 -> Angle Conversion1/1  "<delta_aileron_action_rad>"
  Bus Selector/3 -> Angle Conversion2/1  "<delta_elevator_action_rad>"
  Bus Creator1/1 -> Bus Creator/1  "NonLinear_deltaControls_deg_lbs"

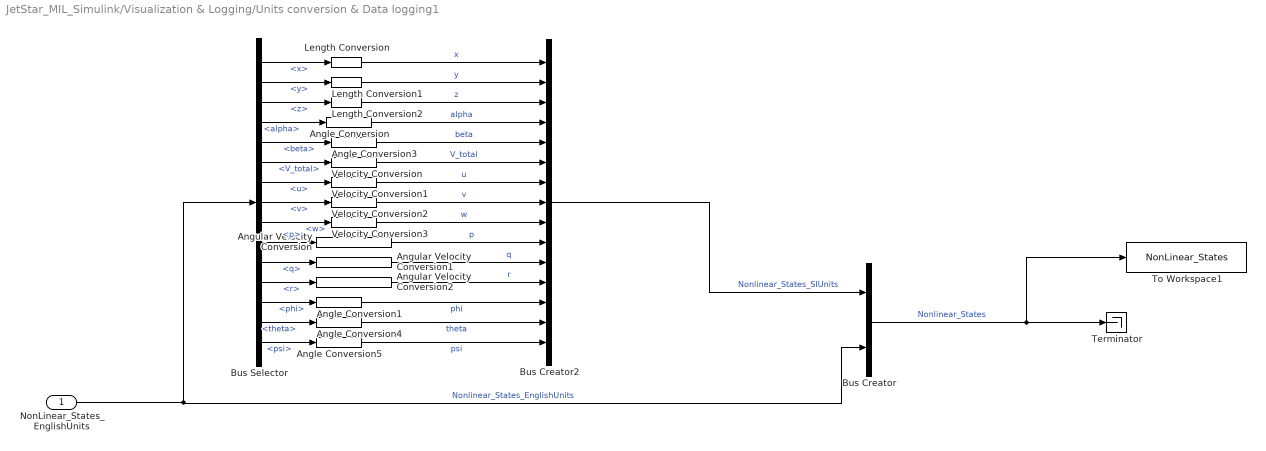
== system JetStar_MIL_Simulink/Visualization & Logging/Units conversion & Data logging1 ==
  NonLinear_States_EnglishUnits : Inport
  Angle Conversion{,1,3..5} (5 alike) : aerolibconvert2/Angle Conversion  IU=rad  OU=deg
  Angular Velocity Conversion : aerolibconvert2/Angular Velocity Conversion  IU=rad/s  OU=deg/s
  Angular Velocity Conversion1 : aerolibconvert2/Angular Velocity Conversion  IU=rad/s  OU=deg/s
  Angular Velocity Conversion2 : aerolibconvert2/Angular Velocity Conversion  IU=rad/s  OU=deg/s
  Bus Creator : BusCreator  Inputs=2
  Bus Creator2 : BusCreator  Inputs=15
  Bus Selector : BusSelector  OutputSignals=x,y,z,alpha,beta,V_total,u,v,w,p,q,r,phi,theta,psi
  Length Conversion : aerolibconvert2/Length Conversion  IU=ft  OU=m
  Length Conversion1 : aerolibconvert2/Length Conversion  IU=ft  OU=m
  Length Conversion2 : aerolibconvert2/Length Conversion  IU=ft  OU=m
  Terminator : Terminator
  To Workspace1 : ToWorkspace  VariableName=NonLinear_States  SaveFormat=Timeseries  SampleTime=-1
  Velocity Conversion{,1..3} (4 alike) : aerolibconvert2/Velocity Conversion  IU=ft/s  OU=m/s
  wires:
  NonLinear_States_EnglishUnits/1 -> Bus Selector/1, Bus Creator/2  "Nonlinear_States_EnglishUnits"
  Bus Creator/1 -> Terminator/1, To Workspace1/1  "Nonlinear_States"
  Bus Selector/1 -> Length Conversion/1  "<x>"
  Bus Selector/2 -> Length Conversion1/1  "<y>"
  Bus Selector/3 -> Length Conversion2/1  "<z>"
  Bus Selector/4 -> Angle Conversion/1  "<alpha>"
  Bus Selector/5 -> Angle Conversion3/1  "<beta>"
  Bus Selector/6 -> Velocity Conversion/1  "<V_total>"
  Bus Selector/7 -> Velocity Conversion1/1  "<u>"
  Bus Selector/8 -> Velocity Conversion2/1  "<v>"
  Bus Selector/9 -> Velocity Conversion3/1  "<w>"
  Bus Selector/10 -> Angular Velocity Conversion/1  "<p>"
  Bus Selector/11 -> Angular Velocity Conversion1/1  "<q>"
  Bus Selector/12 -> Angular Velocity Conversion2/1  "<r>"
  Bus Selector/13 -> Angle Conversion1/1  "<phi>"
  Bus Selector/14 -> Angle Conversion4/1  "<theta>"
  Bus Selector/15 -> Angle Conversion5/1  "<psi>"
  Length Conversion/1 -> Bus Creator2/1  "x"
  Length Conversion1/1 -> Bus Creator2/2  "y"
  Length Conversion2/1 -> Bus Creator2/3  "z"
  Angle Conversion/1 -> Bus Creator2/4  "alpha"
  Angle Conversion3/1 -> Bus Creator2/5  "beta"
  Velocity Conversion/1 -> Bus Creator2/6  "V_total"
  Velocity Conversion1/1 -> Bus Creator2/7  "u"
  Velocity Conversion2/1 -> Bus Creator2/8  "v"
  Velocity Conversion3/1 -> Bus Creator2/9  "w"
  Angular Velocity Conversion/1 -> Bus Creator2/10  "p"
  Angular Velocity Conversion1/1 -> Bus Creator2/11  "q"
  Angular Velocity Conversion2/1 -> Bus Creator2/12  "r"
  Angle Conversion1/1 -> Bus Creator2/13  "phi"
  Angle Conversion4/1 -> Bus Creator2/14  "theta"
  Angle Conversion5/1 -> Bus Creator2/15  "psi"
  Bus Creator2/1 -> Bus Creator/1  "Nonlinear_States_SIUnits"

== system JetStar_MIL_Simulink/Visualization & Logging/Units conversion & Data logging2 ==
  Linear_deltaControls_rad : Inport
  Angle Conversion : aerolibconvert2/Angle Conversion  IU=rad  OU=deg
  Angle Conversion1 : aerolibconvert2/Angle Conversion  IU=rad  OU=deg
  Angle Conversion2 : aerolibconvert2/Angle Conversion  IU=rad  OU=deg
  Bus Creator : BusCreator  Inputs=2
  Bus Creator1 : BusCreator  Inputs=4
  Bus Selector : BusSelector  OutputSignals=delta_rudder_action_rad,delta_aileron_action_rad,delta_elevator_action_rad,delta_thrust_action_lbs
  Gain : Gain
  Terminator : Terminator
  To Workspace : ToWorkspace  VariableName=Linear_deltaControls  SaveFormat=Timeseries  SampleTime=-1
  wires:
  Angle Conversion2/1 -> Bus Creator1/3  "delta_elevator_action_deg"
  Linear_deltaControls_rad/1 -> Bus Selector/1, Bus Creator/2  "Linear_deltaControls_rad_lbs"
  Angle Conversion1/1 -> Bus Creator1/2  "delta_aileron_action_deg"
  Angle Conversion/1 -> Bus Creator1/1  "delta_rudder_action_deg"
  Bus Selector/1 -> Angle Conversion/1  "<delta_rudder_action_rad>"
  Bus Selector/4 -> Gain/1  "<delta_thrust_action_lbs>"
  Bus Creator/1 -> To Workspace/1, Terminator/1  "Linear_deltaControls"
  Gain/1 -> Bus Creator1/4  "delta_thrust_action_lbs"
  Bus Selector/2 -> Angle Conversion1/1  "<delta_aileron_action_rad>"
  Bus Selector/3 -> Angle Conversion2/1  "<delta_elevator_action_rad>"
  Bus Creator1/1 -> Bus Creator/1  "Linear_deltaControls_deg_lbs"

== system JetStar_MIL_Simulink/Visualization & Logging/Units conversion & Data logging3 ==
  Linear_DeltaStates_EnglishUnits : Inport
  Angle Conversion : aerolibconvert2/Angle Conversion  IU=rad  OU=deg
  Angle Conversion3 : aerolibconvert2/Angle Conversion  IU=rad  OU=deg
  Angular Velocity Conversion : aerolibconvert2/Angular Velocity Conversion  IU=rad/s  OU=deg/s
  Angular Velocity Conversion1 : aerolibconvert2/Angular Velocity Conversion  IU=rad/s  OU=deg/s
  Bus Creator : BusCreator  Inputs=2
  Bus Creator2 : BusCreator  Inputs=7
  Bus Selector : BusSelector  OutputSignals=delta_p_radsec,delta_r_radsec,delta_phi_rad,delta_psi_rad,delta_v,delta_u,delta_w
  Terminator : Terminator
  To Workspace1 : ToWorkspace  VariableName=Linear_deltaStates  SaveFormat=Timeseries  SampleTime=-1
  Velocity Conversion : aerolibconvert2/Velocity Conversion  IU=ft/s  OU=m/s
  Velocity Conversion4 : aerolibconvert2/Velocity Conversion  IU=ft/s  OU=m/s
  Velocity Conversion5 : aerolibconvert2/Velocity Conversion  IU=ft/s  OU=m/s
  wires:
  Linear_DeltaStates_EnglishUnits/1 -> Bus Selector/1, Bus Creator/2  "Linear_DeltaStates_EnglishUnits"
  Bus Creator/1 -> Terminator/1, To Workspace1/1  "Linear_DeltaStates"
  Bus Creator2/1 -> Bus Creator/1  "Linear_DeltaStates_SIUnits"
  Bus Selector/1 -> Angular Velocity Conversion/1  "<delta_p_radsec>"
  Bus Selector/2 -> Angular Velocity Conversion1/1  "<delta_r_radsec>"
  Bus Selector/3 -> Angle Conversion/1  "<delta_phi_rad>"
  Bus Selector/4 -> Angle Conversion3/1  "<delta_psi_rad>"
  Bus Selector/5 -> Velocity Conversion/1  "<delta_v>"
  Bus Selector/6 -> Velocity Conversion4/1  "<delta_u>"
  Bus Selector/7 -> Velocity Conversion5/1  "<delta_w>"
  Angular Velocity Conversion/1 -> Bus Creator2/1  "delta_p_degsec"
  Angular Velocity Conversion1/1 -> Bus Creator2/2  "delta_r_degsec"
  Angle Conversion/1 -> Bus Creator2/3  "delta_phi_degsec"
  Angle Conversion3/1 -> Bus Creator2/4  "delta_psi_deg"
  Velocity Conversion/1 -> Bus Creator2/5  "delta_v"
  Velocity Conversion4/1 -> Bus Creator2/6  "delta_u"
  Velocity Conversion5/1 -> Bus Creator2/7  "delta_w"

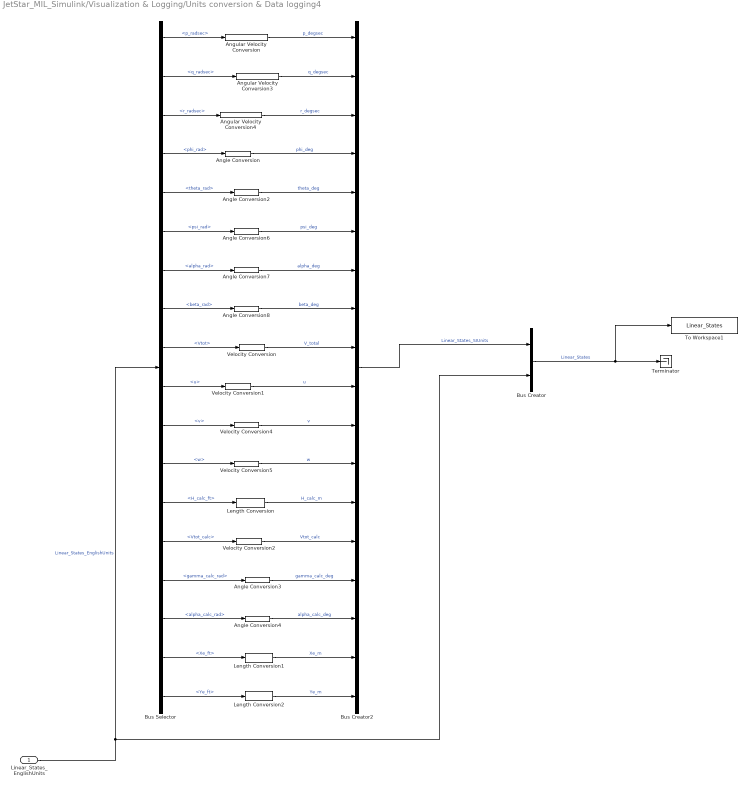
== system JetStar_MIL_Simulink/Visualization & Logging/Units conversion & Data logging4 ==
  Linear_States_EnglishUnits : Inport
  Angle Conversion{,2..4,6..8} (7 alike) : aerolibconvert2/Angle Conversion  IU=rad  OU=deg
  Angular Velocity Conversion : aerolibconvert2/Angular Velocity Conversion  IU=rad/s  OU=deg/s
  Angular Velocity Conversion3 : aerolibconvert2/Angular Velocity Conversion  IU=rad/s  OU=deg/s
  Angular Velocity Conversion4 : aerolibconvert2/Angular Velocity Conversion  IU=rad/s  OU=deg/s
  Bus Creator : BusCreator  Inputs=2
  Bus Creator2 : BusCreator  Inputs=18
  Bus Selector : BusSelector  OutputSignals=p_radsec,q_radsec,r_radsec,phi_rad,theta_rad,psi_rad,alpha_rad,beta_rad,Vtot,u,v,w,H_calc_ft,Vtot_calc,gamma_calc_rad,alpha_calc_rad,Xe_ft,Ye_ft
  Length Conversion : aerolibconvert2/Length Conversion  IU=ft  OU=m
  Length Conversion1 : aerolibconvert2/Length Conversion  IU=ft  OU=m
  Length Conversion2 : aerolibconvert2/Length Conversion  IU=ft  OU=m
  Terminator : Terminator
  To Workspace1 : ToWorkspace  VariableName=Linear_States  SaveFormat=Timeseries  SampleTime=-1
  Velocity Conversion{,1..2,4..5} (5 alike) : aerolibconvert2/Velocity Conversion  IU=ft/s  OU=m/s
  wires:
  Bus Creator2/1 -> Bus Creator/1  "Linear_States_SIUnits"
  Bus Creator/1 -> To Workspace1/1, Terminator/1  "Linear_States"
  Linear_States_EnglishUnits/1 -> Bus Selector/1, Bus Creator/2  "Linear_States_EnglishUnits"
  Bus Selector/5 -> Angle Conversion2/1  "<theta_rad>"
  Bus Selector/6 -> Angle Conversion6/1  "<psi_rad>"
  Bus Selector/1 -> Angular Velocity Conversion/1  "<p_radsec>"
  Bus Selector/2 -> Angular Velocity Conversion3/1  "<q_radsec>"
  Bus Selector/3 -> Angular Velocity Conversion4/1  "<r_radsec>"
  Bus Selector/4 -> Angle Conversion/1  "<phi_rad>"
  Bus Selector/7 -> Angle Conversion7/1  "<alpha_rad>"
  Bus Selector/8 -> Angle Conversion8/1  "<beta_rad>"
  Bus Selector/9 -> Velocity Conversion/1  "<Vtot>"
  Bus Selector/10 -> Velocity Conversion1/1  "<u>"
  Bus Selector/11 -> Velocity Conversion4/1  "<v>"
  Bus Selector/12 -> Velocity Conversion5/1  "<w>"
  Angular Velocity Conversion/1 -> Bus Creator2/1  "p_degsec"
  Angular Velocity Conversion3/1 -> Bus Creator2/2  "q_degsec"
  Angular Velocity Conversion4/1 -> Bus Creator2/3  "r_degsec"
  Angle Conversion/1 -> Bus Creator2/4  "phi_deg"
  Angle Conversion2/1 -> Bus Creator2/5  "theta_deg"
  Angle Conversion6/1 -> Bus Creator2/6  "psi_deg"
  Angle Conversion7/1 -> Bus Creator2/7  "alpha_deg"
  Angle Conversion8/1 -> Bus Creator2/8  "beta_deg"
  Velocity Conversion/1 -> Bus Creator2/9  "V_total"
  Velocity Conversion1/1 -> Bus Creator2/10  "u"
  Velocity Conversion4/1 -> Bus Creator2/11  "v"
  Velocity Conversion5/1 -> Bus Creator2/12  "w"
  Bus Selector/13 -> Length Conversion/1  "<H_calc_ft>"
  Bus Selector/14 -> Velocity Conversion2/1  "<Vtot_calc>"
  Bus Selector/15 -> Angle Conversion3/1  "<gamma_calc_rad>"
  Bus Selector/16 -> Angle Conversion4/1  "<alpha_calc_rad>"
  Bus Selector/17 -> Length Conversion1/1  "<Xe_ft>"
  Bus Selector/18 -> Length Conversion2/1  "<Ye_ft>"
  Length Conversion/1 -> Bus Creator2/13  "H_calc_m"
  Velocity Conversion2/1 -> Bus Creator2/14  "Vtot_calc"
  Angle Conversion3/1 -> Bus Creator2/15  "gamma_calc_deg"
  Angle Conversion4/1 -> Bus Creator2/16  "alpha_calc_deg"
  Length Conversion1/1 -> Bus Creator2/17  "Xe_m"
  Length Conversion2/1 -> Bus Creator2/18  "Ye_m"

== system JetStar_MIL_Simulink/Visualization & Logging/Units conversion & Data logging5 ==
  Command_EnglishUnits : Inport
  Angle Conversion : aerolibconvert2/Angle Conversion  IU=rad  OU=deg
  Angle Conversion1 : aerolibconvert2/Angle Conversion  IU=rad  OU=deg
  Angle Conversion2 : aerolibconvert2/Angle Conversion  IU=rad  OU=deg
  Angular Velocity Conversion : aerolibconvert2/Angular Velocity Conversion  IU=rad/s  OU=deg/s
  Bus Creator : BusCreator  Inputs=6
  Bus Creator1 : BusCreator  Inputs=2
  Bus Selector : BusSelector  OutputSignals=delta_aileron_comm,H_Command,Psi_Command_rad,Phi_Comm,Delta_U_comm,r_comm
  Length Conversion : aerolibconvert2/Length Conversion  IU=ft  OU=m
  To Workspace5 : ToWorkspace  VariableName=Command  SaveFormat=Timeseries  SampleTime=-1
  Velocity Conversion : aerolibconvert2/Velocity Conversion  IU=ft/s  OU=m/s
  wires:
  Angle Conversion/1 -> Bus Creator/1  "delta_aileron_comm"
  Bus Selector/3 -> Angle Conversion1/1  "<Psi_Command_rad>"
  Bus Creator1/1 -> To Workspace5/1  "Commands"
  Velocity Conversion/1 -> Bus Creator/5  "Delta_U_comm"
  Command_EnglishUnits/1 -> Bus Selector/1, Bus Creator1/1
  Bus Selector/2 -> Length Conversion/1  "<H_Command>"
  Bus Selector/4 -> Angle Conversion2/1  "<Phi_Comm>"
  Bus Selector/1 -> Angle Conversion/1  "<delta_aileron_comm>"
  Bus Creator/1 -> Bus Creator1/2  "Command_SIUnits"
  Angle Conversion2/1 -> Bus Creator/4  "Phi_Comm"
  Angular Velocity Conversion/1 -> Bus Creator/6  "r_comm"
  Angle Conversion1/1 -> Bus Creator/3  "Psi_Command_deg"
  Bus Selector/5 -> Velocity Conversion/1  "<Delta_U_comm>"
  Bus Selector/6 -> Angular Velocity Conversion/1  "<r_comm>"
  Length Conversion/1 -> Bus Creator/2  "H_Command"

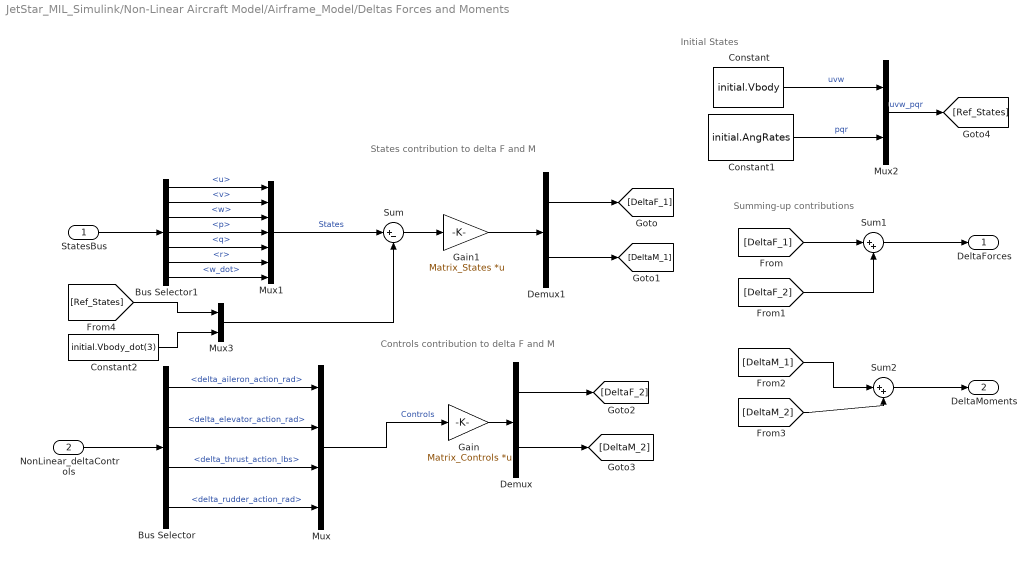
== system JetStar_MIL_Simulink/Non-Linear Aircraft Model/Airframe_Model/Deltas Forces and Moments ==
  note: Initial States
  note: Summing-up contributions
  note: Controls contribution
      |  to delta F and M
  note: States contribution to delta F and M
  StatesBus : Inport  OutDataTypeStr=Bus: Nonlinear_States_Bus
  NonLinear_deltaControls : Inport  Port=2  OutDataTypeStr=Bus: Nonlinear_ControlsAction_Bus
  Bus Selector : BusSelector  OutputSignals=delta_aileron_action_rad,delta_elevator_action_rad,delta_thrust_action_lbs,delta_rudder_action_rad
  Bus Selector1 : BusSelector  OutputSignals=u,v,w,p,q,r,w_dot
  Constant : Constant  Value=initial.Vbody
  Constant1 : Constant  Value=initial.AngRates
  Constant2 : Constant  Value=initial.Vbody_dot(3)
  Demux : Demux  Outputs=2
  Demux1 : Demux  Outputs=2
  Gain : Gain  Gain=Matrix_Controls  Multiplication=Matrix(K*u)
  Gain1 : Gain  Gain=Matrix_States  Multiplication=Matrix(K*u)
  Mux : Mux
  Mux1 : Mux  Inputs=7
  Mux2 : Mux  Inputs=2
  Mux3 : Mux  Inputs=2
  Sum : Sum  Inputs=|+-
  Sum1 : Sum  Inputs=|++
  Sum2 : Sum  Inputs=|++
  DeltaForces : Outport
  DeltaMoments : Outport  Port=2
  wires:
  StatesBus/1 -> Bus Selector1/1
  Demux1/1 -> [DeltaF_1]
  Demux1/2 -> [DeltaM_1]
  Sum/1 -> Gain1/1
  Mux1/1 -> Sum/1  "States"
  Gain1/1 -> Demux1/1
  Mux/1 -> Gain/1  "Controls"
  Demux/1 -> [DeltaF_2]
  Demux/2 -> [DeltaM_2]
  Gain/1 -> Demux/1
  Mux2/1 -> [Ref_States]  "uvw_pqr"
  Constant1/1 -> Mux2/2  "pqr"
  Constant/1 -> Mux2/1  "uvw"
  [DeltaF_1] -> Sum1/1
  [DeltaF_2] -> Sum1/2
  Sum1/1 -> DeltaForces/1
  [DeltaM_1] -> Sum2/1
  [DeltaM_2] -> Sum2/2
  Sum2/1 -> DeltaMoments/1
  Bus Selector1/1 -> Mux1/1  "<u>"
  Bus Selector1/2 -> Mux1/2  "<v>"
  Bus Selector1/3 -> Mux1/3  "<w>"
  Bus Selector1/4 -> Mux1/4  "<p>"
  Bus Selector1/5 -> Mux1/5  "<q>"
  Bus Selector1/6 -> Mux1/6  "<r>"
  Bus Selector1/7 -> Mux1/7  "<w_dot>"
  [Ref_States] -> Mux3/1
  Constant2/1 -> Mux3/2
  Mux3/1 -> Sum/2
  NonLinear_deltaControls/1 -> Bus Selector/1
  Bus Selector/1 -> Mux/1  "<delta_aileron_action_rad>"
  Bus Selector/2 -> Mux/2  "<delta_elevator_action_rad>"
  Bus Selector/3 -> Mux/3  "<delta_thrust_action_lbs>"
  Bus Selector/4 -> Mux/4  "<delta_rudder_action_rad>"

== system JetStar_MIL_Simulink/Non-Linear Aircraft Model/Euler_6DOF/Gravity Force ==
  note: Gravity Transformation
  DCM : Inport
  Gain : Gain  Commented=on  Gain=[0;0;Vehicle.Airframe.mass*g]  Multiplication=Matrix(u*K)
  Gain3 : Gain  Gain=Vehicle.Airframe.mass
  "Gravity Earth " : Constant  Value=[0;0;g]  VectorParams1D=off
  MatrixMultiply : Product  Multiplication=Matrix(*)
  Signal Specification : SignalSpecification  Dimensions=[3 1]
  Gravity_body : Outport
  wires:
  Signal Specification/1 -> Gravity_body/1
  MatrixMultiply/1 -> Signal Specification/1
  "Gravity Earth "/1 -> Gain3/1
  DCM/1 -> MatrixMultiply/1
  Gain3/1 -> MatrixMultiply/2

== matlab function JetStar_MIL_Simulink/Linear_DeltaStates 2 Linear States/MATLAB Function ==
  data: u_v_w input; Xe_dot output; phi_theta_psi input; Ye_dot output; Ze_dot output
function [Xe_dot , Ye_dot, Ze_dot] = fcn(u_v_w, phi_theta_psi)

phi = phi_theta_psi(1);
theta = phi_theta_psi(2);
psi = phi_theta_psi(3);
u = u_v_w(1);
v = u_v_w(2);
w = u_v_w(3);
Transformation_matrix = [
    cos(theta)*cos(psi)   sin(phi)*sin(theta)*cos(psi)-cos(phi)*sin(psi)  cos(phi)*sin(theta)*cos(psi)+sin(phi)*sin(psi)
    cos(theta)*sin(psi)   sin(phi)*sin(theta)*sin(psi)+cos(phi)*cos(psi)  cos(phi)*sin(theta)*sin(psi)-sin(phi)*cos(psi)
    -sin(theta)           sin(phi)*cos(theta)                             cos(phi)*cos(theta)     
    ];
vel_vec = [u;v;w];
Xe_Ye_Ze_dot = Transformation_matrix*vel_vec;
Xe_dot = Xe_Ye_Ze_dot(1);
Ye_dot = Xe_Ye_Ze_dot(2); 
Ze_dot = Xe_Ye_Ze_dot(3);
